simulink model "task_3"  (Simulink 8.3)
settings: Solver=ode45  StartTime=0.0  StopTime=0.3  RelTol=1e-3
settings Model: Creator=Admin  LastModifiedBy=andre
settings OptimizationCC: ExpressionDepthLimit=2147483647
settings DebuggingCC: FcnCallInpInsideContextMsg=UseLocalSettings

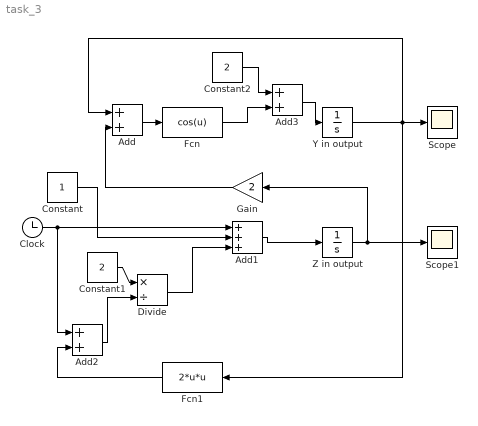
== system task_3 ==
  Add : Sum
  Add1 : Sum  Inputs=+++
  Add2 : Sum
  Add3 : Sum
  Clock : Clock
  Constant : Constant
  Constant1 : Constant  Value=2
  Constant2 : Constant  Value=2
  Divide : Product  Inputs=*/
  Fcn : Fcn  Expr=cos(u)
  Fcn1 : Fcn  Expr=2*u*u
  Gain : Gain  Gain=2
  Scope : Scope
  Scope1 : Scope
  Y in output : Integrator  InitialCondition=1
  Z in output : Integrator  InitialCondition=0.05
  wires:
  Add/1 -> Fcn/1
  Y in output/1 -> Fcn1/1, Add/1, Scope/1
  Z in output/1 -> Gain/1, Scope1/1
  Gain/1 -> Add/2
  Add1/1 -> Z in output/1
  Clock/1 -> Add1/1, Add2/1
  Constant/1 -> Add1/2
  Divide/1 -> Add1/3
  Constant1/1 -> Divide/1
  Add2/1 -> Divide/2
  Fcn1/1 -> Add2/2
  Constant2/1 -> Add3/1
  Fcn/1 -> Add3/2
  Add3/1 -> Y in output/1
